simulink model "gm_DUALportRAMinterface_test"  (R2024a)
settings: Solver=FixedStepDiscrete  StartTime=0.0  StopTime=10  RelTol=1e-3
undefined symbols (not defined in the file or in its folder): Ts
libraries: hdlsllib x34, simulink x1
settings Model: Creator=Simon  LastModifiedBy=Simon
settings OptimizationCC: BlockReduction=off  ConditionallyExecuteInputs=off  DefaultParameterBehavior=Inlined  InheritOutputTypeSmallerThanSingle=on
settings DebuggingCC: AlgebraicLoopMsg=error  InheritedTsInSrcMsg=none  SingleTaskRateTransMsg=error  UnconnectedInputMsg=warning  UnconnectedOutputMsg=warning  UnconnectedLineMsg=warning
settings HardwareCC: ProdBitPerPointer=32  ProdBitPerSizeT=32  ProdBitPerPtrDiffT=32  ProdLargestAtomicFloat=None  ProdIntDivRoundTo=Undefined  ProdEndianess=Unspecified  ProdWordSize=32  ProdHWDeviceType=ASIC/FPGA->ASIC/FPGA  TargetBitPerPointer=64  TargetBitPerSizeT=64  TargetBitPerPtrDiffT=64  TargetLongLongMode=on  TargetIntDivRoundTo=Zero  TargetEndianess=LittleEndian  TargetWordSize=64  TargetHWDeviceType=Custom Processor->MATLAB Host Computer  ProdEqTarget=off

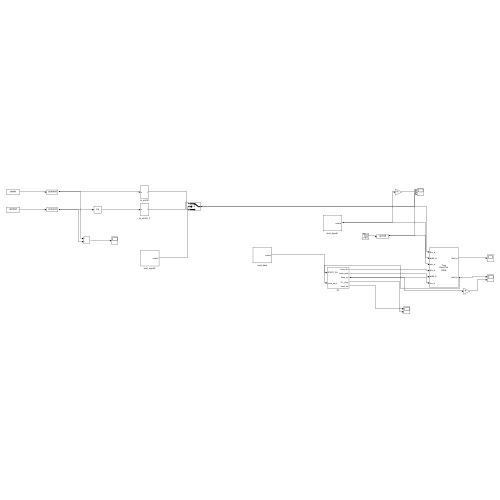
[thumbnail: Simulink's stored preview of the top-level diagram]
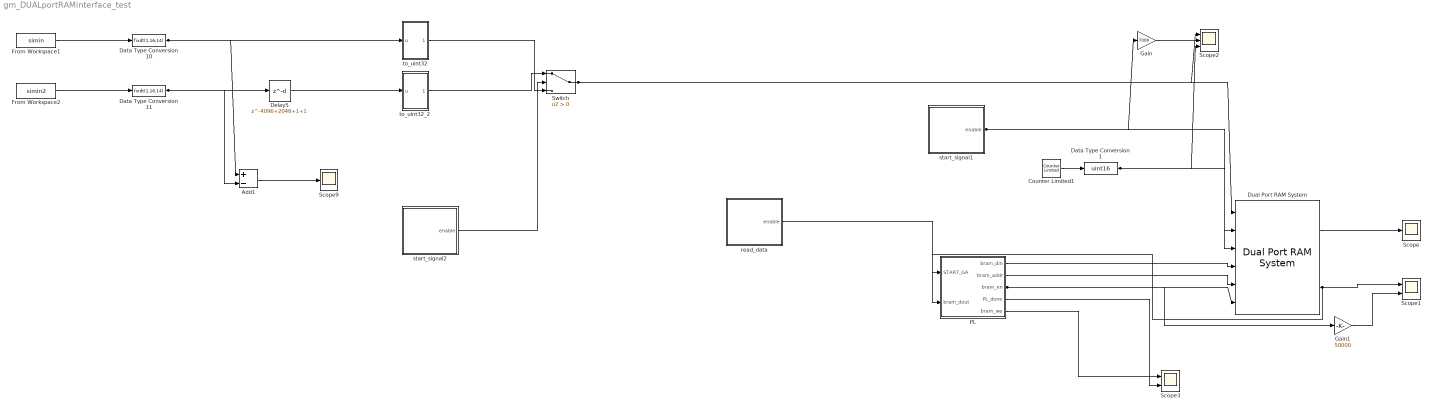
== system gm_DUALportRAMinterface_test ==
  Add1 : Sum  Inputs=+-
  Counter Limited1 : simulink/Sources/Counter Limited  uplimit=14000  tsamp=Ts
  Data Type Conversion1 : DataTypeConversion  OutDataTypeStr=uint16  SaturateOnIntegerOverflow=off  RndMeth=Floor
  Data Type Conversion10 : DataTypeConversion  OutDataTypeStr=fixdt(1,16,14)  SaturateOnIntegerOverflow=off  RndMeth=Floor
  Data Type Conversion11 : DataTypeConversion  OutDataTypeStr=fixdt(1,16,14)  SaturateOnIntegerOverflow=off  RndMeth=Floor
  Delay5 : Delay  DelayLength=4096+2048+1+1  InitialCondition=0  SampleTime=Ts
  Dual Port RAM System : hdlsllib/HDL RAMs/Dual Port RAM System  RAMType=True dual port  AsyncRead=off  WriteOutputValue=New data  RAMInitialValue=0  allowBusInputs=off  WritesHaveOutput=on  NumReads=0  NumWrites=1  SimulateUsing=Code generation
  From Workspace1 : FromWorkspace  VariableName=simin  SampleTime=Ts
  From Workspace2 : FromWorkspace  VariableName=simin2  SampleTime=Ts
  Gain : Gain  Gain=7000
  Gain1 : Gain  Gain=50000
  PL : Subsystem
  Scope : Scope
  Scope1 : Scope  NumInputPorts=2
  Scope2 : Scope  NumInputPorts=3
  Scope3 : Scope  NumInputPorts=2
  Scope9 : Scope
  Switch : Switch  Criteria=u2 > Threshold  SaturateOnIntegerOverflow=off  InputSameDT=off  OutDataTypeStr=Inherit: Same as first input
  read_data : Subsystem
  start_signal1 : Subsystem
  start_signal2 : Subsystem
  to_uint32 : Subsystem
  to_uint32_2 : Subsystem
  wires:
  Gain1/1 -> Scope1/2
  PL/5(bram_we) -> Scope3/1
  PL/4(PL_done) -> Scope3/2
  Data Type Conversion10/1 -> to_uint32/1(u), Add1/1
  Add1/1 -> Scope9/1
  Data Type Conversion11/1 -> Add1/2, Delay5/1
  Switch/1 -> Dual Port RAM System/1, Scope2/1
  Delay5/1 -> to_uint32_2/1(u)
  start_signal2/1(enable) -> Switch/2
  to_uint32_2/1(Out1) -> Switch/1
  to_uint32/1(Out1) -> Switch/3
  From Workspace2/1 -> Data Type Conversion11/1
  From Workspace1/1 -> Data Type Conversion10/1
  Dual Port RAM System/2 -> PL/2(bram_dout), Scope1/1
  read_data/1(enable) -> PL/1(START_GA)
  Gain/1 -> Scope2/2
  PL/3(bram_en) -> Dual Port RAM System/6, Gain1/1
  PL/2(bram_addr) -> Dual Port RAM System/5
  PL/1(bram_din) -> Dual Port RAM System/4
  start_signal1/1(enable) -> Gain/1, Dual Port RAM System/3
  Data Type Conversion1/1 -> Dual Port RAM System/2, Scope2/3
  Counter Limited1/1 -> Data Type Conversion1/1
  Dual Port RAM System/1 -> Scope/1

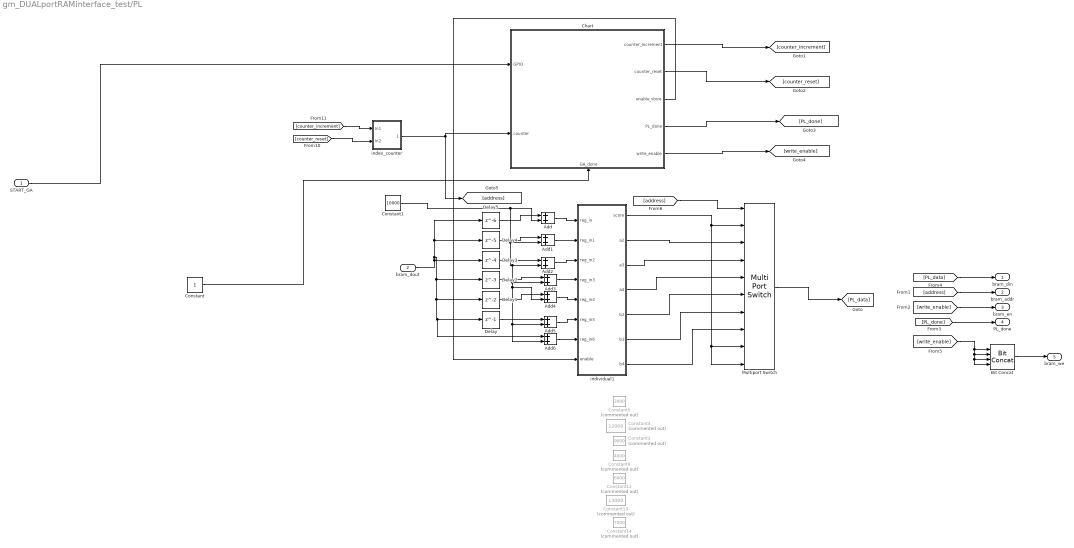
== system gm_DUALportRAMinterface_test/PL ==
  START_GA : Inport
  bram_dout : Inport  Port=2
  Add{,1..6} (7 alike) : Sum  OutDataTypeStr=Inherit: Same as first input
  Bit Concat : hdlsllib/Logic and Bit Operations/Bit Concat  numInputs=4
  Chart : Stateflow chart  TreatAsAtomicUnit=on
      settings: PortSchema="{\"entries\":[{\"content\":{\"sides\":[{\"content\":{\"connectorIds\":[\"In2\",\"In3\"]},\"type\":\"ConnectorPlacement.EquallySpacedRectSide\",\"uuid\":\"f3ce331f-c708-4668-a9cb-fb327ea74ab5\"},{\"content\":{\"connectorIds\":[\"Out1\",\"Out2\",\"Out3\",\"Out4\",\"Out5\"],\"side\":\"RIGHT\"},\"type\":\"ConnectorPlacement.EquallySpacedRectSide\",\"uuid\":\"3766927a-abff-497d-9544-2098881ba174\"},{\"content\":{\"side\":\"TOP\"},\"type\":\"ConnectorPlacement.EquallySpacedRectSide\",\"uuid\":\"ebfe3d64-ee7d-4953-a6ba-e7e40988decf\"},{\"content\":{\"connectorIds\":[\"In1\"],\"side\":\"BOTTOM\"},\"type\":\"ConnectorPlacement.EquallySpacedRectSide\",\"uuid\":\"f39ceaf8-4df7-4e40-9de5-da7597831fb4\"}]},\"type\":\"ConnectorPlacement.EquallySpacedConnector\",\"uuid\":\"89f60450-5933-42bb-b72b-5f8ec55483e0\"}],\"packageUris\":[\"http://schema.mathworks.com/mf0/Connector/R2020b\"],\"version\":\"1.0\"}"
  Constant : Constant  OutDataTypeStr=boolean  SampleTime=-1
  Constant1 : Constant  Value=10000  OutDataTypeStr=uint32  SampleTime=-1
  Constant12 : Constant  Commented=on  Value=6000  OutDataTypeStr=uint32  SampleTime=Ts
  Constant13 : Constant  Commented=on  Value=13000  OutDataTypeStr=uint32  SampleTime=Ts
  Constant14 : Constant  Commented=on  Value=7000  OutDataTypeStr=uint32  SampleTime=Ts
  Constant3 : Constant  Commented=on  Value=9000  OutDataTypeStr=uint32  SampleTime=Ts
  Constant4 : Constant  Commented=on  Value=12000  OutDataTypeStr=uint32  SampleTime=Ts
  Constant5 : Constant  Commented=on  Value=2000  OutDataTypeStr=uint32  SampleTime=Ts
  Constant9 : Constant  Commented=on  Value=4000  OutDataTypeStr=uint32  SampleTime=Ts
  Delay : Delay  DelayLength=1  InitialCondition=0
  Delay1 : Delay  InitialCondition=0
  Delay2 : Delay  DelayLength=3  InitialCondition=0
  Delay3 : Delay  DelayLength=4  InitialCondition=0
  Delay4 : Delay  DelayLength=5  InitialCondition=0
  Delay5 : Delay  DelayLength=6  InitialCondition=0
  Multiport Switch : MultiPortSwitch  DataPortOrder=Specify indices  Inputs=8  DataPortIndices={0,1,2,3,4,5,6,7}  DataPortForDefault=Additional data port  DiagnosticForDefault=None  OutDataTypeStr=Inherit: Same as first data input  SaturateOnIntegerOverflow=off  InputSameDT=off
  index_counter : Subsystem
  individual1 : Subsystem
  bram_din : Outport
  bram_addr : Outport  Port=2
  bram_en : Outport  Port=3
  PL_done : Outport  Port=4
  bram_we : Outport  Port=5
  wires:
  Add6/1 -> individual1/7(reg_in6)
  Add5/1 -> individual1/6(reg_in5)
  Add4/1 -> individual1/5(reg_in4)
  Add3/1 -> individual1/4(reg_in3)
  Add2/1 -> individual1/3(reg_in2)
  Add1/1 -> individual1/2(reg_in1)
  Add/1 -> individual1/1(reg_in)
  Constant1/1 -> Add/2, Add1/2, Add2/2, Add3/2, Add4/2, Add5/2, Add6/2
  Delay5/1 -> Add/1
  Delay4/1 -> Add1/1
  Delay3/1 -> Add2/1
  Delay2/1 -> Add3/1
  Delay1/1 -> Add4/1
  Delay/1 -> Add5/1
  Chart/3(enable_store) -> individual1/8(enable)
  Bit Concat/1 -> bram_we/1
  [write_enable] -> Bit Concat/1, Bit Concat/2, Bit Concat/3, Bit Concat/4
  Chart/4(PL_done) -> [PL_done]
  [PL_done] -> PL_done/1
  bram_dout/1 -> Delay3/1, Delay4/1, Delay5/1, Delay2/1, Delay1/1, Delay/1, Add6/1
  individual1/7(b4) -> Multiport Switch/8
  individual1/6(b3) -> Multiport Switch/7
  individual1/5(b2) -> Multiport Switch/6
  individual1/4(a4) -> Multiport Switch/5
  individual1/3(a3) -> Multiport Switch/4
  individual1/2(a2) -> Multiport Switch/3
  individual1/1(score) -> Multiport Switch/2, Multiport Switch/9, Multiport Switch/10
  [write_enable] -> bram_en/1
  [PL_data] -> bram_din/1
  Chart/1(counter_increment) -> [counter_increment]
  Chart/2(counter_reset) -> [counter_reset]
  START_GA/1 -> Chart/2(GPIO)
  Constant/1 -> Chart/1(GA_done)
  Chart/5(write_enable) -> [write_enable]
  [address] -> Multiport Switch/1
  [counter_increment] -> index_counter/1(In1)
  [address] -> bram_addr/1
  index_counter/1(index_counter) -> [address], Chart/3(counter)
  [counter_reset] -> index_counter/2(In2)
  Multiport Switch/1 -> [PL_data]

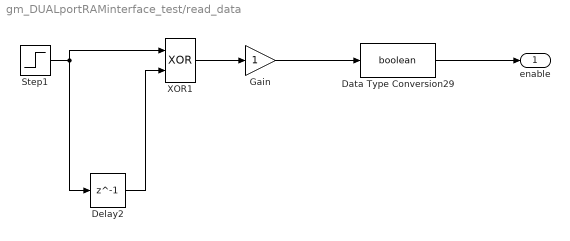
== system gm_DUALportRAMinterface_test/read_data ==
  Data Type Conversion29 : DataTypeConversion  OutDataTypeStr=boolean  SaturateOnIntegerOverflow=off  RndMeth=Floor
  Delay2 : Delay  DelayLength=1  InitialCondition=0  SampleTime=Ts
  Gain : Gain
  Step1 : Step  Time=Ts*14000  SampleTime=Ts
  XOR1 : Logic  Operator=XOR  IconShape=distinctive  AllPortsSameDT=off  OutDataTypeStr=boolean
  enable : Outport
  wires:
  Data Type Conversion29/1 -> enable/1
  Gain/1 -> Data Type Conversion29/1
  Delay2/1 -> XOR1/2
  Step1/1 -> XOR1/1, Delay2/1
  XOR1/1 -> Gain/1

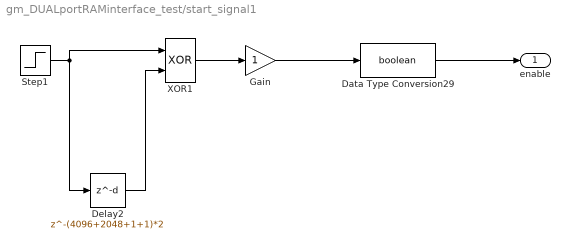
== system gm_DUALportRAMinterface_test/start_signal1 ==
  Data Type Conversion29 : DataTypeConversion  OutDataTypeStr=boolean  SaturateOnIntegerOverflow=off  RndMeth=Floor
  Delay2 : Delay  DelayLength=(4096+2048+1+1)*2  InitialCondition=0  SampleTime=Ts
  Gain : Gain
  Step1 : Step  Time=Ts*0  SampleTime=Ts
  XOR1 : Logic  Operator=XOR  IconShape=distinctive  AllPortsSameDT=off  OutDataTypeStr=boolean
  enable : Outport
  wires:
  XOR1/1 -> Gain/1
  Step1/1 -> Delay2/1, XOR1/1
  Delay2/1 -> XOR1/2
  Gain/1 -> Data Type Conversion29/1
  Data Type Conversion29/1 -> enable/1

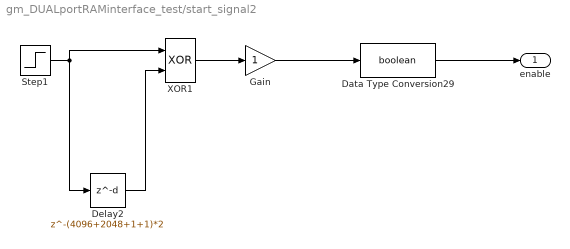
== system gm_DUALportRAMinterface_test/start_signal2 ==
  Data Type Conversion29 : DataTypeConversion  OutDataTypeStr=boolean  SaturateOnIntegerOverflow=off  RndMeth=Floor
  Delay2 : Delay  DelayLength=(4096+2048+1+1)*2  InitialCondition=0  SampleTime=Ts
  Gain : Gain
  Step1 : Step  Time=Ts*(4096+2048+1+1)  SampleTime=Ts
  XOR1 : Logic  Operator=XOR  IconShape=distinctive  AllPortsSameDT=off  OutDataTypeStr=boolean
  enable : Outport
  wires:
  Data Type Conversion29/1 -> enable/1
  Gain/1 -> Data Type Conversion29/1
  Delay2/1 -> XOR1/2
  Step1/1 -> XOR1/1, Delay2/1
  XOR1/1 -> Gain/1

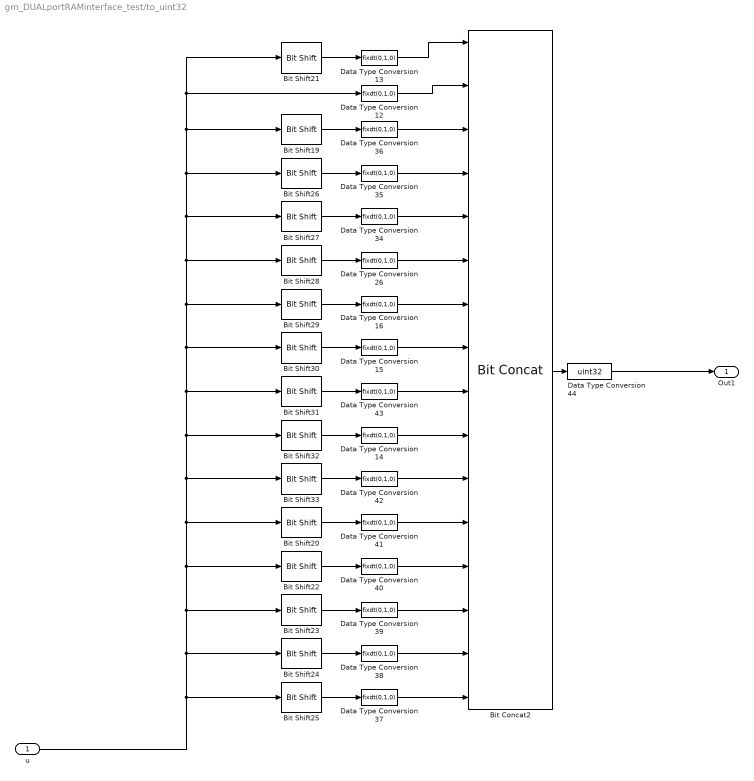
== system gm_DUALportRAMinterface_test/to_uint32 ==
  u : Inport
  Bit Concat2 : hdlsllib/Logic and Bit Operations/Bit Concat  numInputs=16
  Bit Shift19 : hdlsllib/Logic and Bit Operations/Bit Shift  mode=Shift Left Logical  N=1
  Bit Shift20 : hdlsllib/Logic and Bit Operations/Bit Shift  mode=Shift Left Logical  N=10
  Bit Shift21 : hdlsllib/Logic and Bit Operations/Bit Shift  mode=Shift Right Logical  N=1
  Bit Shift22 : hdlsllib/Logic and Bit Operations/Bit Shift  mode=Shift Left Logical  N=11
  Bit Shift23 : hdlsllib/Logic and Bit Operations/Bit Shift  mode=Shift Left Logical  N=12
  Bit Shift24 : hdlsllib/Logic and Bit Operations/Bit Shift  mode=Shift Left Logical  N=13
  Bit Shift25 : hdlsllib/Logic and Bit Operations/Bit Shift  mode=Shift Left Logical  N=14
  Bit Shift26 : hdlsllib/Logic and Bit Operations/Bit Shift  mode=Shift Left Logical  N=2
  Bit Shift27 : hdlsllib/Logic and Bit Operations/Bit Shift  mode=Shift Left Logical  N=3
  Bit Shift28 : hdlsllib/Logic and Bit Operations/Bit Shift  mode=Shift Left Logical  N=4
  Bit Shift29 : hdlsllib/Logic and Bit Operations/Bit Shift  mode=Shift Left Logical  N=5
  Bit Shift30 : hdlsllib/Logic and Bit Operations/Bit Shift  mode=Shift Left Logical  N=6
  Bit Shift31 : hdlsllib/Logic and Bit Operations/Bit Shift  mode=Shift Left Logical  N=7
  Bit Shift32 : hdlsllib/Logic and Bit Operations/Bit Shift  mode=Shift Left Logical  N=8
  Bit Shift33 : hdlsllib/Logic and Bit Operations/Bit Shift  mode=Shift Left Logical  N=9
  Data Type Conversion{12..16,26,34..43} (16 alike) : DataTypeConversion  OutDataTypeStr=fixdt(0,1,0)  SaturateOnIntegerOverflow=off  RndMeth=Floor
  Data Type Conversion44 : DataTypeConversion  OutDataTypeStr=uint32  SaturateOnIntegerOverflow=off  RndMeth=Floor
  Out1 : Outport
  wires:
  Data Type Conversion14/1 -> Bit Concat2/10
  Bit Concat2/1 -> Data Type Conversion44/1
  Bit Shift26/1 -> Data Type Conversion35/1
  Bit Shift21/1 -> Data Type Conversion13/1
  Bit Shift28/1 -> Data Type Conversion26/1
  Data Type Conversion37/1 -> Bit Concat2/16
  Bit Shift29/1 -> Data Type Conversion16/1
  Bit Shift23/1 -> Data Type Conversion39/1
  Data Type Conversion41/1 -> Bit Concat2/12
  Bit Shift24/1 -> Data Type Conversion38/1
  Bit Shift33/1 -> Data Type Conversion42/1
  Data Type Conversion16/1 -> Bit Concat2/7
  Data Type Conversion43/1 -> Bit Concat2/9
  Data Type Conversion34/1 -> Bit Concat2/5
  Data Type Conversion39/1 -> Bit Concat2/14
  Bit Shift32/1 -> Data Type Conversion14/1
  Data Type Conversion12/1 -> Bit Concat2/2
  Bit Shift30/1 -> Data Type Conversion15/1
  Data Type Conversion15/1 -> Bit Concat2/8
  Bit Shift25/1 -> Data Type Conversion37/1
  Data Type Conversion38/1 -> Bit Concat2/15
  Bit Shift19/1 -> Data Type Conversion36/1
  Data Type Conversion42/1 -> Bit Concat2/11
  Data Type Conversion35/1 -> Bit Concat2/4
  Data Type Conversion44/1 -> Out1/1
  Data Type Conversion26/1 -> Bit Concat2/6
  Bit Shift31/1 -> Data Type Conversion43/1
  Data Type Conversion40/1 -> Bit Concat2/13
  Data Type Conversion13/1 -> Bit Concat2/1
  Bit Shift20/1 -> Data Type Conversion41/1
  u/1 -> Bit Shift25/1, Bit Shift24/1, Bit Shift23/1, Bit Shift22/1, Bit Shift20/1, Bit Shift33/1, Bit Shift32/1, Bit Shift31/1, Bit Shift30/1, Bit Shift29/1, Bit Shift28/1, Bit Shift27/1, Bit Shift26/1, Bit Shift19/1, Data Type Conversion12/1, Bit Shift21/1
  Data Type Conversion36/1 -> Bit Concat2/3
  Bit Shift27/1 -> Data Type Conversion34/1
  Bit Shift22/1 -> Data Type Conversion40/1

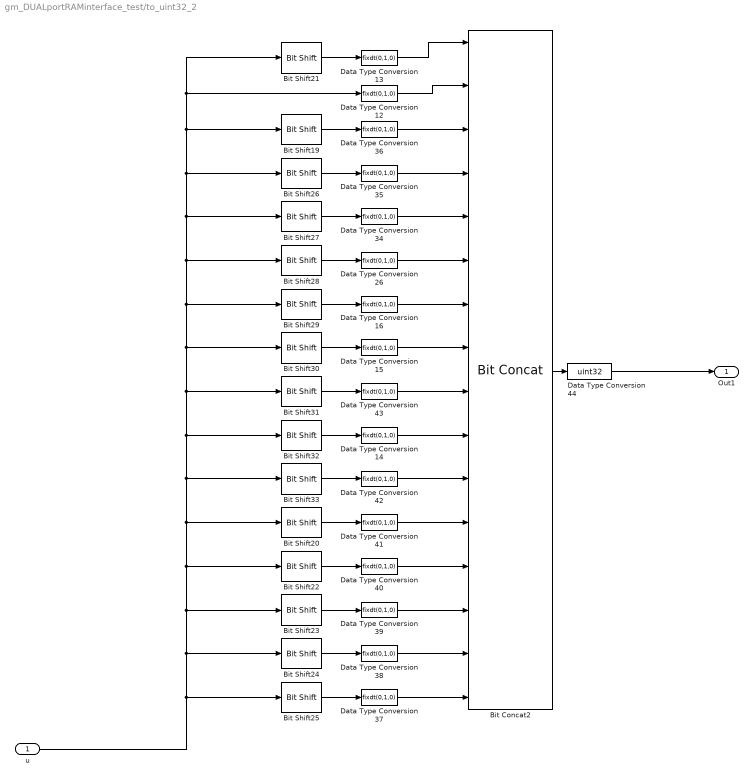
== system gm_DUALportRAMinterface_test/to_uint32_2 ==
  u : Inport
  Bit Concat2 : hdlsllib/Logic and Bit Operations/Bit Concat  numInputs=16
  Bit Shift19 : hdlsllib/Logic and Bit Operations/Bit Shift  mode=Shift Left Logical  N=1
  Bit Shift20 : hdlsllib/Logic and Bit Operations/Bit Shift  mode=Shift Left Logical  N=10
  Bit Shift21 : hdlsllib/Logic and Bit Operations/Bit Shift  mode=Shift Right Logical  N=1
  Bit Shift22 : hdlsllib/Logic and Bit Operations/Bit Shift  mode=Shift Left Logical  N=11
  Bit Shift23 : hdlsllib/Logic and Bit Operations/Bit Shift  mode=Shift Left Logical  N=12
  Bit Shift24 : hdlsllib/Logic and Bit Operations/Bit Shift  mode=Shift Left Logical  N=13
  Bit Shift25 : hdlsllib/Logic and Bit Operations/Bit Shift  mode=Shift Left Logical  N=14
  Bit Shift26 : hdlsllib/Logic and Bit Operations/Bit Shift  mode=Shift Left Logical  N=2
  Bit Shift27 : hdlsllib/Logic and Bit Operations/Bit Shift  mode=Shift Left Logical  N=3
  Bit Shift28 : hdlsllib/Logic and Bit Operations/Bit Shift  mode=Shift Left Logical  N=4
  Bit Shift29 : hdlsllib/Logic and Bit Operations/Bit Shift  mode=Shift Left Logical  N=5
  Bit Shift30 : hdlsllib/Logic and Bit Operations/Bit Shift  mode=Shift Left Logical  N=6
  Bit Shift31 : hdlsllib/Logic and Bit Operations/Bit Shift  mode=Shift Left Logical  N=7
  Bit Shift32 : hdlsllib/Logic and Bit Operations/Bit Shift  mode=Shift Left Logical  N=8
  Bit Shift33 : hdlsllib/Logic and Bit Operations/Bit Shift  mode=Shift Left Logical  N=9
  Data Type Conversion{12..16,26,34..43} (16 alike) : DataTypeConversion  OutDataTypeStr=fixdt(0,1,0)  SaturateOnIntegerOverflow=off  RndMeth=Floor
  Data Type Conversion44 : DataTypeConversion  OutDataTypeStr=uint32  SaturateOnIntegerOverflow=off  RndMeth=Floor
  Out1 : Outport
  wires:
  Bit Shift22/1 -> Data Type Conversion40/1
  Bit Shift27/1 -> Data Type Conversion34/1
  Data Type Conversion36/1 -> Bit Concat2/3
  u/1 -> Bit Shift21/1, Data Type Conversion12/1, Bit Shift19/1, Bit Shift26/1, Bit Shift27/1, Bit Shift28/1, Bit Shift29/1, Bit Shift30/1, Bit Shift31/1, Bit Shift32/1, Bit Shift33/1, Bit Shift20/1, Bit Shift22/1, Bit Shift23/1, Bit Shift24/1, Bit Shift25/1
  Bit Shift20/1 -> Data Type Conversion41/1
  Data Type Conversion13/1 -> Bit Concat2/1
  Data Type Conversion40/1 -> Bit Concat2/13
  Bit Shift31/1 -> Data Type Conversion43/1
  Data Type Conversion26/1 -> Bit Concat2/6
  Data Type Conversion44/1 -> Out1/1
  Data Type Conversion35/1 -> Bit Concat2/4
  Data Type Conversion42/1 -> Bit Concat2/11
  Bit Shift19/1 -> Data Type Conversion36/1
  Data Type Conversion38/1 -> Bit Concat2/15
  Bit Shift25/1 -> Data Type Conversion37/1
  Data Type Conversion15/1 -> Bit Concat2/8
  Bit Shift30/1 -> Data Type Conversion15/1
  Data Type Conversion12/1 -> Bit Concat2/2
  Bit Shift32/1 -> Data Type Conversion14/1
  Data Type Conversion39/1 -> Bit Concat2/14
  Data Type Conversion34/1 -> Bit Concat2/5
  Data Type Conversion43/1 -> Bit Concat2/9
  Data Type Conversion16/1 -> Bit Concat2/7
  Bit Shift33/1 -> Data Type Conversion42/1
  Bit Shift24/1 -> Data Type Conversion38/1
  Data Type Conversion41/1 -> Bit Concat2/12
  Bit Shift23/1 -> Data Type Conversion39/1
  Bit Shift29/1 -> Data Type Conversion16/1
  Data Type Conversion37/1 -> Bit Concat2/16
  Bit Shift28/1 -> Data Type Conversion26/1
  Bit Shift21/1 -> Data Type Conversion13/1
  Bit Shift26/1 -> Data Type Conversion35/1
  Bit Concat2/1 -> Data Type Conversion44/1
  Data Type Conversion14/1 -> Bit Concat2/10

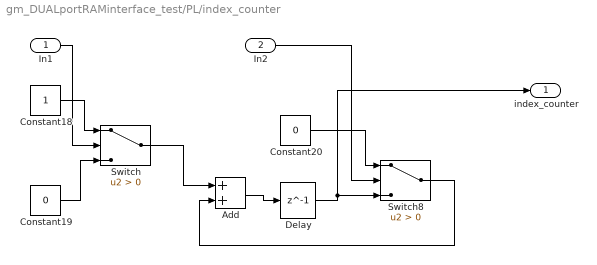
== system gm_DUALportRAMinterface_test/PL/index_counter ==
  In1 : Inport
  In2 : Inport  Port=2
  Add : Sum  OutDataTypeStr=Inherit: Same as first input
  Constant18 : Constant  OutDataTypeStr=fixdt(0,16,0)  SampleTime=Ts
  Constant19 : Constant  Value=0  OutDataTypeStr=fixdt(0,16,0)  SampleTime=Ts
  Constant20 : Constant  Value=0  OutDataTypeStr=uint16  SampleTime=Ts
  Delay : Delay  DelayLength=1  InitialCondition=0  SampleTime=Ts
  Switch : Switch  Criteria=u2 > Threshold  SaturateOnIntegerOverflow=off  InputSameDT=off  OutDataTypeStr=Inherit: Same as first input
  Switch8 : Switch  Criteria=u2 > Threshold  SaturateOnIntegerOverflow=off  InputSameDT=off  OutDataTypeStr=Inherit: Same as first input
  index_counter : Outport
  wires:
  In1/1 -> Switch/2
  Constant18/1 -> Switch/1
  Constant20/1 -> Switch8/1
  Add/1 -> Delay/1
  In2/1 -> Switch8/2
  Delay/1 -> Switch8/3, index_counter/1
  Switch/1 -> Add/1
  Switch8/1 -> Add/2
  Constant19/1 -> Switch/3

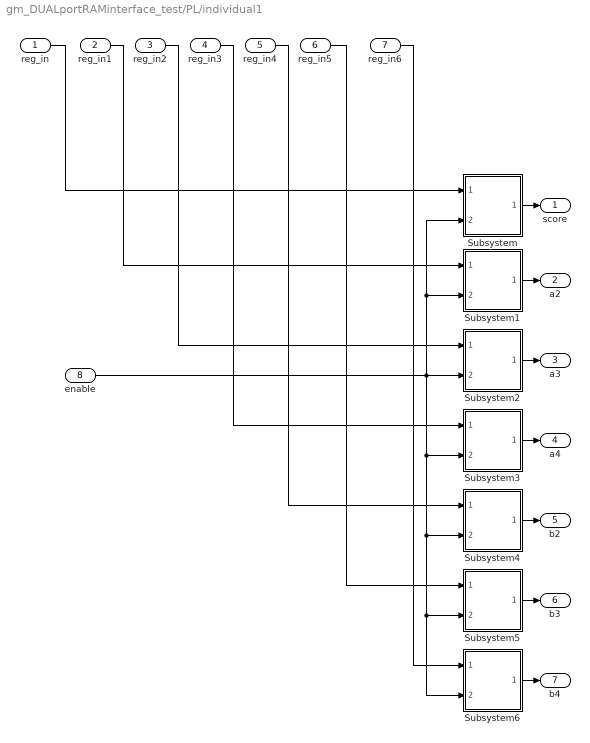
== system gm_DUALportRAMinterface_test/PL/individual1 ==
  reg_in : Inport
  reg_in1 : Inport  Port=2
  reg_in2 : Inport  Port=3
  reg_in3 : Inport  Port=4
  reg_in4 : Inport  Port=5
  reg_in5 : Inport  Port=6
  reg_in6 : Inport  Port=7
  enable : Inport  Port=8
  Subsystem : Subsystem
  Subsystem1 : Subsystem
  Subsystem2 : Subsystem
  Subsystem3 : Subsystem
  Subsystem4 : Subsystem
  Subsystem5 : Subsystem
  Subsystem6 : Subsystem
  score : Outport
  a2 : Outport  Port=2
  a3 : Outport  Port=3
  a4 : Outport  Port=4
  b2 : Outport  Port=5
  b3 : Outport  Port=6
  b4 : Outport  Port=7
  wires:
  reg_in6/1 -> Subsystem6/1(reg_in)
  Subsystem6/1(reg_out) -> b4/1
  reg_in5/1 -> Subsystem5/1(reg_in)
  reg_in4/1 -> Subsystem4/1(reg_in)
  Subsystem5/1(reg_out) -> b3/1
  reg_in3/1 -> Subsystem3/1(reg_in)
  reg_in2/1 -> Subsystem2/1(reg_in)
  reg_in1/1 -> Subsystem1/1(reg_in)
  Subsystem/1(reg_out) -> score/1
  reg_in/1 -> Subsystem/1(reg_in)
  Subsystem1/1(reg_out) -> a2/1
  Subsystem3/1(reg_out) -> a4/1
  Subsystem4/1(reg_out) -> b2/1
  Subsystem2/1(reg_out) -> a3/1
  enable/1 -> Subsystem/2(enable), Subsystem1/2(enable), Subsystem2/2(enable), Subsystem6/2(enable), Subsystem5/2(enable), Subsystem4/2(enable), Subsystem3/2(enable)

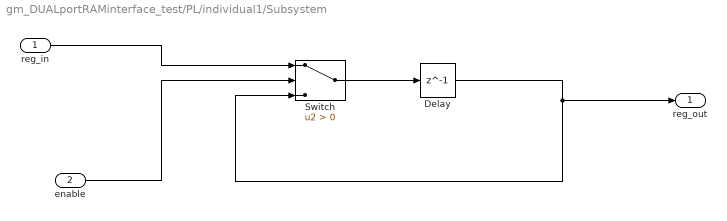
== system gm_DUALportRAMinterface_test/PL/individual1/Subsystem ==
  reg_in : Inport
  enable : Inport  Port=2
  Delay : Delay  DelayLength=1  InitialCondition=0  SampleTime=Ts
  Switch : Switch  Criteria=u2 > Threshold  SaturateOnIntegerOverflow=off  InputSameDT=off  OutDataTypeStr=Inherit: Same as first input
  reg_out : Outport  OutDataTypeStr=uint32
  wires:
  reg_in/1 -> Switch/1
  enable/1 -> Switch/2
  Switch/1 -> Delay/1
  Delay/1 -> Switch/3, reg_out/1

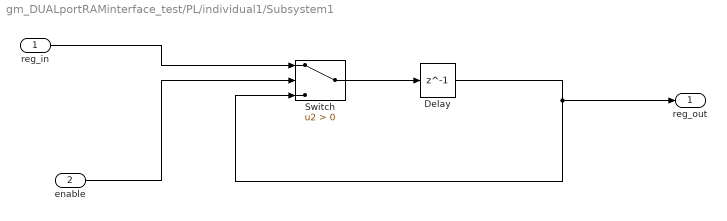
== system gm_DUALportRAMinterface_test/PL/individual1/Subsystem1 ==
  reg_in : Inport
  enable : Inport  Port=2
  Delay : Delay  DelayLength=1  InitialCondition=0  SampleTime=Ts
  Switch : Switch  Criteria=u2 > Threshold  SaturateOnIntegerOverflow=off  InputSameDT=off  OutDataTypeStr=Inherit: Same as first input
  reg_out : Outport
  wires:
  reg_in/1 -> Switch/1
  enable/1 -> Switch/2
  Switch/1 -> Delay/1
  Delay/1 -> Switch/3, reg_out/1

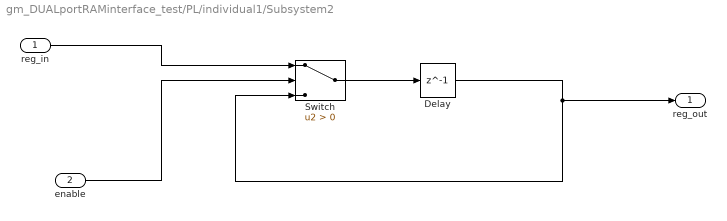
== system gm_DUALportRAMinterface_test/PL/individual1/Subsystem2 ==
  reg_in : Inport
  enable : Inport  Port=2
  Delay : Delay  DelayLength=1  InitialCondition=0  SampleTime=Ts
  Switch : Switch  Criteria=u2 > Threshold  SaturateOnIntegerOverflow=off  InputSameDT=off  OutDataTypeStr=Inherit: Same as first input
  reg_out : Outport
  wires:
  reg_in/1 -> Switch/1
  enable/1 -> Switch/2
  Switch/1 -> Delay/1
  Delay/1 -> Switch/3, reg_out/1

== system gm_DUALportRAMinterface_test/PL/individual1/Subsystem3 ==
  reg_in : Inport
  enable : Inport  Port=2
  Delay : Delay  DelayLength=1  InitialCondition=0  SampleTime=Ts
  Switch : Switch  Criteria=u2 > Threshold  SaturateOnIntegerOverflow=off  InputSameDT=off  OutDataTypeStr=Inherit: Same as first input
  reg_out : Outport
  wires:
  reg_in/1 -> Switch/1
  enable/1 -> Switch/2
  Switch/1 -> Delay/1
  Delay/1 -> Switch/3, reg_out/1

== system gm_DUALportRAMinterface_test/PL/individual1/Subsystem4 ==
  reg_in : Inport
  enable : Inport  Port=2
  Delay : Delay  DelayLength=1  InitialCondition=0  SampleTime=Ts
  Switch : Switch  Criteria=u2 > Threshold  SaturateOnIntegerOverflow=off  InputSameDT=off  OutDataTypeStr=Inherit: Same as first input
  reg_out : Outport
  wires:
  reg_in/1 -> Switch/1
  enable/1 -> Switch/2
  Switch/1 -> Delay/1
  Delay/1 -> Switch/3, reg_out/1

== system gm_DUALportRAMinterface_test/PL/individual1/Subsystem5 ==
  reg_in : Inport
  enable : Inport  Port=2
  Delay : Delay  DelayLength=1  InitialCondition=0  SampleTime=Ts
  Switch : Switch  Criteria=u2 > Threshold  SaturateOnIntegerOverflow=off  InputSameDT=off  OutDataTypeStr=Inherit: Same as first input
  reg_out : Outport
  wires:
  reg_in/1 -> Switch/1
  enable/1 -> Switch/2
  Switch/1 -> Delay/1
  Delay/1 -> Switch/3, reg_out/1

== system gm_DUALportRAMinterface_test/PL/individual1/Subsystem6 ==
  reg_in : Inport
  enable : Inport  Port=2
  Delay : Delay  DelayLength=1  InitialCondition=0  SampleTime=Ts
  Switch : Switch  Criteria=u2 > Threshold  SaturateOnIntegerOverflow=off  InputSameDT=off  OutDataTypeStr=Inherit: Same as first input
  reg_out : Outport
  wires:
  Delay/1 -> reg_out/1, Switch/3
  Switch/1 -> Delay/1
  enable/1 -> Switch/2
  reg_in/1 -> Switch/1

== stateflow chart gm_DUALportRAMinterface_test/PL/Chart ==
  settings: executeAtInitialization=1
  state initial_wait_state
    entry:
    counter_increment = false;
    counter_reset = true;
    write_enable = false;
    PL_done = false;
    enable_store = false;
  state PL_read_data
    entry:
    counter_increment = true;
    counter_reset = false;
    write_enable = false;
    PL_done = false;
    enable_store = true;
  state wait_for_GA_done
    entry:
    counter_increment = false;
    counter_reset = true;
    write_enable = false;
    PL_done = false;
    enable_store = false;
  state reset_state
    entry:
    counter_increment = false;
    counter_reset = true;
    write_enable = false;
    PL_done = true;
    enable_store = false;
  state PL_write_data_back
    entry:
    counter_increment = true;
    counter_reset = false;
    write_enable = true;
    PL_done = false;
    enable_store = false;
  (default) -> initial_wait_state
  initial_wait_state -> PL_read_data : [GPIO == 1]
  PL_read_data -> wait_for_GA_done : [counter == (4096+2048+1)*2]
  wait_for_GA_done -> PL_write_data_back : [GA_done == 1]
  PL_write_data_back -> reset_state : [counter == 8]
  data: GA_done input boolean; GPIO input; counter input; counter_increment output boolean; counter_reset output boolean; enable_store output boolean; PL_done output boolean; write_enable output boolean
